simulink model "uz_mpc_6ph"  (R2021a)
settings: Solver=FixedStepDiscrete  StartTime=0.0  StopTime=3*1/f  RelTol=1e-3
values from neighbouring files (symbols this model uses):
  A = 1.0    (= 1)    [uz_6ph_pu_vsd_voltages_init.m]    (also in uz_mpc_6ph_init.m; uz_mpc_6ph_state_machine_init.m = 0.1)
  f = n_rpm/60.0*p    (= 250)    [uz_6ph_pu_vsd_voltages_init.m]    (also in uz_mpc_6ph_init.m; uz_mpc_6ph_state_machine_init.m = 83.3333333333)
  IB = sqrt(2)*IR    [uz_6ph_pu_vsd_voltages_init.m]    (also in uz_mpc_6ph_init.m; uz_mpc_6ph_state_machine_init.m)
  id_ref = 0.0    (= 0)    [uz_6ph_pu_vsd_voltages_init.m]    (also in uz_mpc_6ph_init.m; uz_mpc_6ph_state_machine_init.m)
  iq_ref = -10.0    (= -10)    [uz_6ph_pu_vsd_voltages_init.m]    (also in uz_mpc_6ph_init.m; uz_mpc_6ph_state_machine_init.m = 5)
  ix_ref = 0.0    (= 0)    [uz_6ph_pu_vsd_voltages_init.m]    (also in uz_mpc_6ph_init.m; uz_mpc_6ph_state_machine_init.m)
  iy_ref = 0.0    (= 0)    [uz_6ph_pu_vsd_voltages_init.m]    (also in uz_mpc_6ph_init.m; uz_mpc_6ph_state_machine_init.m)
  Ld_minus_Lq_over_LB = (Ld-Lq)/LB    [uz_6ph_pu_vsd_voltages_init.m]    (also in uz_mpc_6ph_init.m; uz_mpc_6ph_state_machine_init.m)
  Ld_over_LB = Ld/LB    [uz_6ph_pu_vsd_voltages_init.m]    (also in uz_mpc_6ph_init.m; uz_mpc_6ph_state_machine_init.m)
  Lq_over_LB = Lq/LB    [uz_6ph_pu_vsd_voltages_init.m]    (also in uz_mpc_6ph_init.m; uz_mpc_6ph_state_machine_init.m)
  omega_m = n_rpm*pi/30    (= 314.159265359)    [uz_6ph_pu_vsd_voltages_init.m]    (also in uz_mpc_6ph_init.m; uz_mpc_6ph_state_machine_init.m = 104.71975512)
  omegaB = nR*2*pi()/60*p    [uz_6ph_pu_vsd_voltages_init.m]    (also in uz_mpc_6ph_init.m; uz_mpc_6ph_state_machine_init.m)
  psi_pm_over_psiB = psi_pm/psiB    [uz_6ph_pu_vsd_voltages_init.m]    (also in uz_mpc_6ph_init.m; uz_mpc_6ph_state_machine_init.m)
  Rs_over_ZB = Rs/ZB    [uz_6ph_pu_vsd_voltages_init.m]    (also in uz_mpc_6ph_init.m; uz_mpc_6ph_state_machine_init.m)
  t_ADC = 1/f_ADC    (= 1e-05)    [uz_6ph_pu_vsd_voltages_init.m]    (also in uz_mpc_6ph_init.m; uz_mpc_6ph_state_machine_init.m; uz_typeconv_init.m)
  Ts_times_ZB_over_Ld = Ts*ZB/Ld    [uz_6ph_pu_vsd_voltages_init.m]    (also in uz_mpc_6ph_init.m; uz_mpc_6ph_state_machine_init.m)
  Ts_times_ZB_over_Lq = Ts*ZB/Lq    [uz_6ph_pu_vsd_voltages_init.m]    (also in uz_mpc_6ph_init.m; uz_mpc_6ph_state_machine_init.m)
  Ts_times_ZB_over_Lx = Ts*ZB/Lx    [uz_6ph_pu_vsd_voltages_init.m]    (also in uz_mpc_6ph_init.m; uz_mpc_6ph_state_machine_init.m)
  Ts_times_ZB_over_Ly = Ts*ZB/Ly    [uz_6ph_pu_vsd_voltages_init.m]    (also in uz_mpc_6ph_init.m; uz_mpc_6ph_state_machine_init.m)
  v_dc = 565.0    (= 565)    [uz_6ph_pu_vsd_voltages_init.m]    (also in uz_mpc_6ph_init.m; uz_mpc_6ph_state_machine_init.m)
  VB = sqrt(2/3)*VR    [uz_6ph_pu_vsd_voltages_init.m]    (also in uz_mpc_6ph_init.m; uz_mpc_6ph_state_machine_init.m)
libraries: fl_lib x7, nesl_utility x7, simulink x4, ee_lib x2, hdlsllib x1
(part 1 of 2)
settings Model: DataTypeOverride=Off  Creator=micha  LastModifiedBy=micha
settings SolverCC: AlgebraicLoopSolver=TrustRegion
settings DataIOCC: LimitDataPoints=on  SaveOutput=off  SaveTime=off
settings OptimizationCC: BlockReduction=off  ConditionallyExecuteInputs=off  DefaultParameterBehavior=Inlined  LifeSpan=inf
settings DebuggingCC: SignalRangeChecking=warning  AlgebraicLoopMsg=error  SingleTaskRateTransMsg=error  AllowSymbolicDim=off  StrictBusMsg=ErrorOnBusTreatedAsVector  SFUnexpectedBacktrackingDiag=warning  SFNoUnconditionalDefaultTransitionDiag=warning  SFExecutionAtInitializationDiag=none  SFMachineParentedDataDiag=warning  ArithmeticOperatorsInVariantConditions=warning
settings HardwareCC: ProdBitPerPointer=32  ProdBitPerSizeT=32  ProdBitPerPtrDiffT=32  ProdLargestAtomicFloat=None  ProdIntDivRoundTo=Undefined  ProdEndianess=Unspecified  ProdWordSize=32  ProdHWDeviceType=ASIC/FPGA->ASIC/FPGA  ProdEqTarget=off
settings SFSimCC: SimUseLocalCustomCode=off  CustomCodeUndefinedFunction=UseInterfaceOnly
settings RTWCC: RTWUseLocalCustomCode=off
settings CodeAppCC: StateflowObjectComments=on
settings GRTTargetCC: TargetLangStandard=C89/C90 (ANSI)
settings ConfigComp: CovScope=ReferencedModels  CovMetricSettings=dw  CovSaveCumulativeToWorkspaceVar=on  CovSaveSingleToWorkspaceVar=on  CovExternalEMLEnable=off  CovSFcnEnable=off

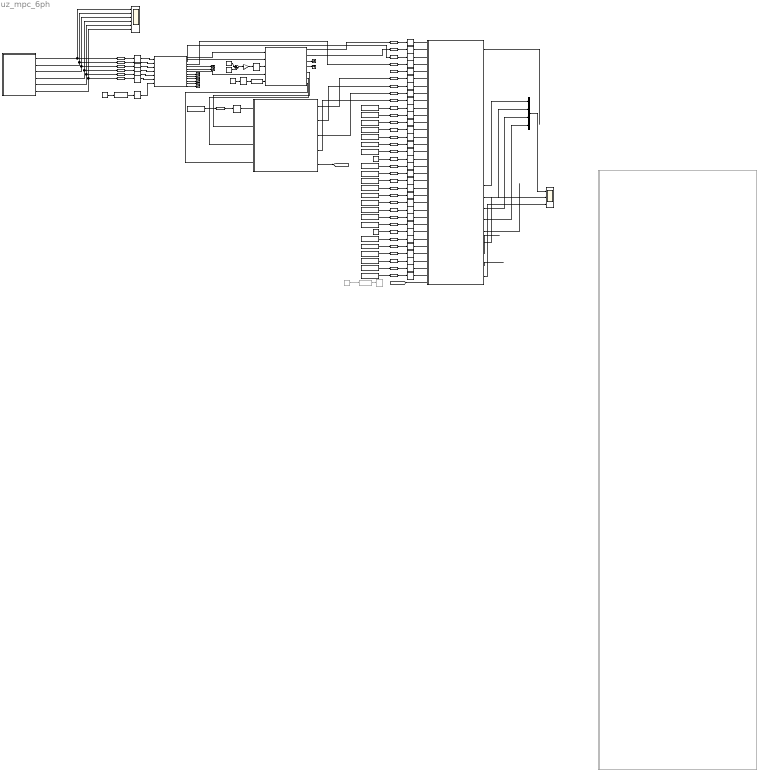
== system uz_mpc_6ph ==
  note: 0=AXI, 1=PL
  Constant : Constant  Value=5
  Constant1 : Constant  Value=0
  Constant10 : Constant  Value=psi_pm_over_psiB
  Constant11 : Constant  Value=2.5
  Constant12 : Constant  Value=0.0
  Constant{13..16} (4 alike) : Constant  Value=1.0
  Constant17 : Constant  Value=v_dc/VB
  Constant18 : Constant  Value=v_dc/VB
  Constant19 : Constant  Value=id_ref/IB
  Constant2 : Constant  Value=Rs_over_ZB
  Constant20 : Constant  Value=iq_ref/IB
  Constant21 : Constant  Value=ix_ref/IB
  Constant22 : Constant  Value=iy_ref/IB
  Constant23 : Constant  Value=omega_m/omegaB
  Constant24 : Constant  Value=2*pi
  Constant25 : Constant
  Constant26 : Constant  Value=v_dc/VB
  Constant3 : Constant  Value=Ts_times_ZB_over_Ld
  Constant4 : Constant  Value=Ts_times_ZB_over_Lq
  Constant5 : Constant  Value=Ts_times_ZB_over_Lx
  Constant6 : Constant  Value=Ts_times_ZB_over_Ly
  Constant7 : Constant  Value=Ld_over_LB
  Constant8 : Constant  Value=Lq_over_LB
  Constant9 : Constant  Value=Ld_minus_Lq_over_LB
  Data Type Conversion{,1,4,8..11} (7 alike) : DataTypeConversion  OutDataTypeStr=fixdt_type_xy_currents
  Data Type Conversion12 : DataTypeConversion  OutDataTypeStr=boolean
  Data Type Conversion13 : DataTypeConversion  OutDataTypeStr=fixdt_type_polepairs
  Data Type Conversion{14..18} (5 alike) : DataTypeConversion  OutDataTypeStr=fixdt_type_lambda
  Data Type Conversion19 : DataTypeConversion  OutDataTypeStr=fixdt_type_max_current
  Data Type Conversion2 : DataTypeConversion  OutDataTypeStr=fixdt_type_dq_currents
  Data Type Conversion{20..28} (9 alike) : DataTypeConversion  OutDataTypeStr=fixdt_type_constants
  Data Type Conversion29 : DataTypeConversion  OutDataTypeStr=fixdt_type_speed
  Data Type Conversion3 : DataTypeConversion  OutDataTypeStr=fixdt_type_dq_currents
  Data Type Conversion30 : DataTypeConversion  OutDataTypeStr=fixdt_type_voltage
  Data Type Conversion31 : DataTypeConversion  OutDataTypeStr=fixdt_type_voltage
  Data Type Conversion{32..36,38} (6 alike) : DataTypeConversion  OutDataTypeStr=fixdt_type_vsd
  Data Type Conversion37 : DataTypeConversion  OutDataTypeStr=boolean
  Data Type Conversion39 : DataTypeConversion  OutDataTypeStr=fixdt(1,18,14)
  Data Type Conversion40 : DataTypeConversion  OutDataTypeStr=fixdt_type_voltage
  Data Type Conversion{6..7,41..42} (4 alike) : DataTypeConversion  OutDataTypeStr=fixdt_type_dqxy_voltages
  Data Type Conversion5 : DataTypeConversion  Commented=on  OutDataTypeStr=boolean
  Gain : Gain  Gain=0.5
  Mux : Mux
  Pulse Generator : DiscretePulseGenerator  Commented=on  PulseType=Time based  Period=t_ADC  PulseWidth=5
  Pulse Generator1 : DiscretePulseGenerator  PulseType=Time based  Period=t_ADC  PulseWidth=5
  Rate Transition{1..2,4..43,58} (43 alike) : RateTransition  OutPortSampleTime=t_clock
  Rate Transition3 : RateTransition  Commented=on  OutPortSampleTime=t_clock
  Sawtooth Generator : SignalGenerator  WaveForm=sawtooth  Amplitude=2*pi  Frequency=2*pi*f  Units=rad/sec
  Scope : Scope  NumInputPorts=3
  Subsystem : Subsystem
  Sum : Sum  Inputs=|+-
  Terminator{,1..9} (10 alike) : Terminator
  natural values : Scope  NumInputPorts=6
  uz_6ph_pu_voltages_vsd : Subsystem
  uz_mpc_6ph : Subsystem  TreatAsAtomicUnit=on
  uz_mpc_current : MATLAB Function  Commented=on  TreatAsAtomicUnit=on  VariantControl=(default)
  uz_park_transformation : Subsystem  TreatAsAtomicUnit=on
  uz_vsd_6ph_30deg : Subsystem  TreatAsAtomicUnit=on
  wires:
  uz_mpc_6ph/1(G_T1) -> ?
  Pulse Generator/1 -> Data Type Conversion5/1
  Data Type Conversion5/1 -> Rate Transition3/1
  [calc_done] -> uz_mpc_6ph/34(trigger)  "trigger"
  Data Type Conversion/1 -> Rate Transition39/1
  Rate Transition39/1 -> uz_mpc_6ph/3(ix_pu)
  Data Type Conversion1/1 -> Rate Transition1/1
  Data Type Conversion2/1 -> Rate Transition2/1
  Data Type Conversion3/1 -> Rate Transition4/1
  Rate Transition1/1 -> uz_mpc_6ph/4(iy_pu)
  Rate Transition4/1 -> uz_mpc_6ph/2(iq_pu)
  Rate Transition2/1 -> uz_mpc_6ph/1(id_pu)
  Data Type Conversion4/1 -> Rate Transition5/1
  Rate Transition5/1 -> uz_mpc_6ph/5(angle_el)
  Data Type Conversion6/1 -> Rate Transition6/1
  Rate Transition6/1 -> uz_mpc_6ph/6(vd_pu)
  Data Type Conversion7/1 -> Rate Transition7/1
  Rate Transition7/1 -> uz_mpc_6ph/7(vq_pu)
  Rate Transition8/1 -> uz_mpc_6ph/11(id_ref_pu_AXI)
  Data Type Conversion8/1 -> Rate Transition8/1
  Rate Transition9/1 -> uz_mpc_6ph/12(iq_ref_pu_AXI)
  Data Type Conversion9/1 -> Rate Transition9/1
  Rate Transition10/1 -> uz_mpc_6ph/13(ix_ref_pu_AXI)
  Data Type Conversion10/1 -> Rate Transition10/1
  Rate Transition11/1 -> uz_mpc_6ph/14(iy_ref_pu_AXI)
  Data Type Conversion11/1 -> Rate Transition11/1
  Data Type Conversion12/1 -> Rate Transition12/1
  Rate Transition12/1 -> uz_mpc_6ph/17(v_dc_select_AXI)
  Data Type Conversion13/1 -> Rate Transition13/1
  Rate Transition13/1 -> uz_mpc_6ph/27(polepairs_AXI)
  Data Type Conversion14/1 -> Rate Transition14/1
  Rate Transition14/1 -> uz_mpc_6ph/29(lambda_u_AXI)
  Data Type Conversion15/1 -> Rate Transition15/1
  Rate Transition15/1 -> uz_mpc_6ph/30(lambda_d_AXI)
  Data Type Conversion16/1 -> Rate Transition16/1
  Rate Transition16/1 -> uz_mpc_6ph/31(lambda_q_AXI)
  Data Type Conversion17/1 -> Rate Transition17/1
  Rate Transition17/1 -> uz_mpc_6ph/32(lambda_x_AXI)
  Data Type Conversion18/1 -> Rate Transition18/1
  Rate Transition18/1 -> uz_mpc_6ph/33(lambda_y_AXI)
  Data Type Conversion19/1 -> Rate Transition19/1
  Rate Transition19/1 -> uz_mpc_6ph/28(max_current_pu_AXI)
  Rate Transition20/1 -> uz_mpc_6ph/15(v_dc_pu)
  Rate Transition21/1 -> uz_mpc_6ph/16(v_dc_pu_AXI)
  Rate Transition22/1 -> uz_mpc_6ph/18(Rs_over_ZB_AXI)
  Rate Transition28/1 -> uz_mpc_6ph/26(psi_pm_over_psiB_AXI)
  Rate Transition29/1 -> uz_mpc_6ph/19(Ts_times_ZB_over_Ld_AXI)
  Rate Transition25/1 -> uz_mpc_6ph/25(Ld_minus_Lq_over_LB_AXI)
  Rate Transition24/1 -> uz_mpc_6ph/22(Ts_times_ZB_over_Ly_AXI)
  Rate Transition26/1 -> uz_mpc_6ph/23(Ld_over_LB_AXI)
  Rate Transition30/1 -> uz_mpc_6ph/20(Ts_times_ZB_over_Lq_AXI)
  Rate Transition23/1 -> uz_mpc_6ph/21(Ts_times_ZB_over_Lx_AXI)
  Rate Transition27/1 -> uz_mpc_6ph/24(Lq_over_LB_AXI)
  Data Type Conversion20/1 -> Rate Transition22/1
  Data Type Conversion21/1 -> Rate Transition29/1
  Data Type Conversion22/1 -> Rate Transition30/1
  Data Type Conversion23/1 -> Rate Transition23/1
  Data Type Conversion24/1 -> Rate Transition24/1
  Data Type Conversion25/1 -> Rate Transition26/1
  Data Type Conversion26/1 -> Rate Transition27/1
  Data Type Conversion27/1 -> Rate Transition25/1
  Data Type Conversion28/1 -> Rate Transition28/1
  Data Type Conversion29/1 -> Rate Transition31/1
  Rate Transition31/1 -> uz_mpc_6ph/10(omega_m_pu)
  Data Type Conversion30/1 -> Rate Transition20/1
  Data Type Conversion31/1 -> Rate Transition21/1
  Constant/1 -> Data Type Conversion13/1
  Constant1/1 -> Data Type Conversion12/1
  Constant2/1 -> Data Type Conversion20/1
  Constant3/1 -> Data Type Conversion21/1
  Constant4/1 -> Data Type Conversion22/1
  Constant5/1 -> Data Type Conversion23/1
  Constant6/1 -> Data Type Conversion24/1
  Constant7/1 -> Data Type Conversion25/1
  Constant8/1 -> Data Type Conversion26/1
  Constant9/1 -> Data Type Conversion27/1
  Constant10/1 -> Data Type Conversion28/1
  Constant11/1 -> Data Type Conversion19/1
  Constant12/1 -> Data Type Conversion14/1
  Constant13/1 -> Data Type Conversion15/1
  Constant16/1 -> Data Type Conversion18/1
  Constant15/1 -> Data Type Conversion17/1
  Constant14/1 -> Data Type Conversion16/1
  Constant17/1 -> Data Type Conversion31/1
  Constant18/1 -> Data Type Conversion30/1
  Constant19/1 -> Data Type Conversion8/1
  Constant20/1 -> Data Type Conversion9/1
  Constant22/1 -> Data Type Conversion11/1
  Constant21/1 -> Data Type Conversion10/1
  Constant23/1 -> Data Type Conversion29/1
  Subsystem/1(output) -> natural values/1, Data Type Conversion32/1
  Rate Transition34/1 -> uz_vsd_6ph_30deg/4(a2)
  Subsystem/4(output3) -> Data Type Conversion35/1, natural values/4
  uz_vsd_6ph_30deg/3(x1) -> Data Type Conversion/1
  Data Type Conversion36/1 -> Rate Transition36/1
  Subsystem/2(output1) -> natural values/2, Data Type Conversion33/1
  Subsystem/5(output4) -> Data Type Conversion36/1, natural values/5
  Data Type Conversion37/1 -> Rate Transition58/1
  Data Type Conversion38/1 -> Rate Transition37/1
  Subsystem/6(output5) -> natural values/6, Data Type Conversion38/1
  Data Type Conversion34/1 -> Rate Transition33/1
  Data Type Conversion32/1 -> Rate Transition35/1
  Subsystem/3(output2) -> Data Type Conversion34/1, natural values/3
  Rate Transition32/1 -> uz_vsd_6ph_30deg/2(b1)
  Data Type Conversion35/1 -> Rate Transition34/1
  uz_vsd_6ph_30deg/5(z1) -> Terminator/1
  uz_vsd_6ph_30deg/1(alpha) -> uz_park_transformation/1(u1)
  Data Type Conversion33/1 -> Rate Transition32/1
  uz_vsd_6ph_30deg/6(z2) -> Terminator1/1
  uz_vsd_6ph_30deg/7(vsd_done) -> uz_park_transformation/4(trigger)
  uz_vsd_6ph_30deg/4(y1) -> Data Type Conversion1/1
  uz_vsd_6ph_30deg/2(beta) -> uz_park_transformation/2(u2)
  Rate Transition37/1 -> uz_vsd_6ph_30deg/6(c2)
  Pulse Generator1/1 -> Data Type Conversion37/1
  Rate Transition58/1 -> uz_vsd_6ph_30deg/7(pu_conv_valid)
  Rate Transition35/1 -> uz_vsd_6ph_30deg/1(a1)
  Rate Transition36/1 -> uz_vsd_6ph_30deg/5(b2)
  Rate Transition33/1 -> uz_vsd_6ph_30deg/3(c1)
  uz_6ph_pu_voltages_vsd/5(calc_done) -> [calc_done]  "calc_done"
  uz_park_transformation/1(y1) -> Data Type Conversion2/1
  uz_park_transformation/2(y2) -> Data Type Conversion3/1
  Sawtooth Generator/1 -> Sum/2
  Sum/1 -> Gain/1
  Constant24/1 -> Sum/1
  Gain/1 -> Rate Transition38/1
  Rate Transition38/1 -> uz_park_transformation/3(angle_el)
  Constant25/1 -> Rate Transition40/1
  Rate Transition40/1 -> Data Type Conversion39/1
  Data Type Conversion39/1 -> uz_park_transformation/5(factor_angle_el_AXI)
  Rate Transition41/1 -> uz_6ph_pu_voltages_vsd/1(v_DC_pu)
  Constant26/1 -> Data Type Conversion40/1
  Data Type Conversion40/1 -> Rate Transition41/1
  uz_park_transformation/5(sin) -> uz_6ph_pu_voltages_vsd/2(sin_angle)
  uz_park_transformation/6(cos) -> uz_6ph_pu_voltages_vsd/3(cos_angle)
  uz_park_transformation/7(calc_done) -> uz_6ph_pu_voltages_vsd/4(trigger)  "calc_done"
  Data Type Conversion41/1 -> Rate Transition42/1
  Data Type Conversion42/1 -> Rate Transition43/1
  Rate Transition42/1 -> uz_mpc_6ph/8(vx_pu)
  Rate Transition43/1 -> uz_mpc_6ph/9(vy_pu)
  uz_6ph_pu_voltages_vsd/1(pu_ud) -> Data Type Conversion6/1
  uz_6ph_pu_voltages_vsd/2(pu_uq) -> Data Type Conversion7/1
  uz_6ph_pu_voltages_vsd/3(pu_ux) -> Data Type Conversion41/1
  uz_6ph_pu_voltages_vsd/4(pu_uy) -> Data Type Conversion42/1
  uz_mpc_6ph/13(id_pred_pu_AXI) -> Mux/1
  uz_mpc_6ph/14(iq_pred_pu_AXI) -> Mux/2
  uz_mpc_6ph/15(ix_pred_pu_AXI) -> Mux/3
  uz_mpc_6ph/16(iy_pred_pu_AXI) -> Mux/4
  uz_mpc_6ph/17(T_el_pred_pu_AXI) -> ?
  uz_mpc_6ph/18(index_AXI) -> Scope/2
  uz_mpc_6ph/19(id_delay_pu_AXI) -> ?
  uz_mpc_6ph/20(iq_delay_pu_AXI) -> ?
  Mux/1 -> Scope/1
  uz_mpc_6ph/21(calc_done) -> Scope/3
  uz_vsd_6ph_30deg/8(alpha_AXI) -> Terminator2/1
  uz_vsd_6ph_30deg/9(beta_AXI) -> Terminator3/1
  uz_vsd_6ph_30deg/10(x_AXI) -> Terminator4/1
  uz_vsd_6ph_30deg/11(y_AXI) -> Terminator5/1
  uz_vsd_6ph_30deg/12(z1_AXI) -> Terminator6/1
  uz_vsd_6ph_30deg/13(z2_AXI) -> Terminator7/1
  uz_park_transformation/3(y1_AXI) -> Terminator8/1
  uz_park_transformation/4(y2_AXI) -> Terminator9/1

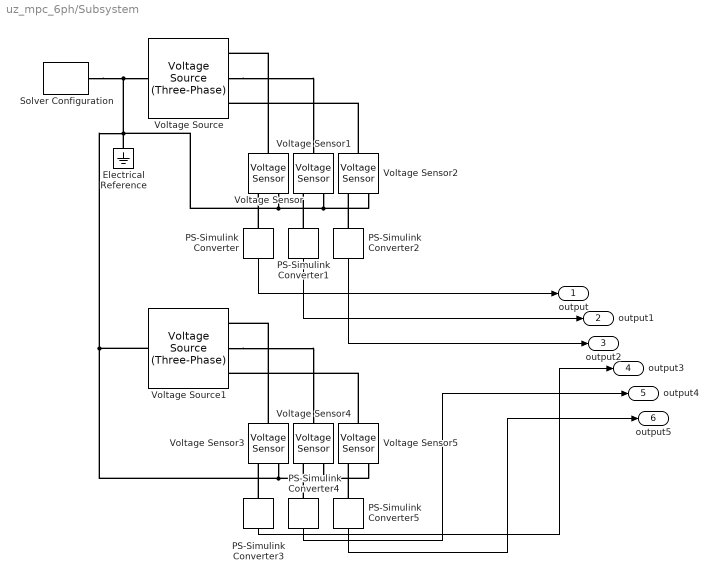
== system uz_mpc_6ph/Subsystem ==
  Electrical Reference : fl_lib/Electrical/Electrical Elements/Electrical Reference
  PS-Simulink Converter{,1..5} (6 alike) : nesl_utility/PS-Simulink Converter  PhysicalDomain=network_engine_domain  SubClassName=ps_output  LeftPortType=input  RightPortType=output  PseudoPeriodic=off  Frequencies=[]  Unit=1  AffineConversion=off
  Solver Configuration : nesl_utility/Solver Configuration  PhysicalDomain=network_engine_domain  SubClassName=solver  LeftPortType=input  RightPortType=generic  Tones=[]  Harmonics=[]  SimulateNoise=off  Profile=off  UseLocalSampling=off  EnableSwitchedLinearOptims=on  FrequencyDomain=off  UseCCode=off  RelTol=0.001  AbsTol=1e-06  MinStep=1e-09  ToWorkspace=off  RevertToSquareIcSolve=off  NumHomotopyIterations=100  PhasorMode=off  PhasorModeNumHarmonics=1  DoDC=off  ResidualTolerance=1e-09  UseLocalSolver=on  LocalSolverChoice=NE_BACKWARD_EULER_ADVANCER  LocalSolverSampleTime=1e-6  DoFixedCost=on  MaxNonlinIter=3  MaxModeIter=2  ComputeImpulses=off  ImpulseIterations=2  LinearAlgebra=Sparse  EquationFormulation=NE_TIME_EF  DelaysMemoryBudget=1024  AutomaticFiltering=on  FilteringTimeConstant=0.001  PartitionStorageMethod=AS_NEEDED  PartitionMemoryBudget=1024  PartitionMethod=FAST
  Voltage Sensor{,1..5} (6 alike) : fl_lib/Electrical/Electrical Sensors/Voltage Sensor
  Voltage Source : ee_lib/Sources/Voltage Source (Three-Phase)  vline_rms=A*sqrt(3)/sqrt(2) V  shift=0 deg  freq=f Hz  impedance_option=1  SShortCircuit=1e6 V*A  XR=15  R=0.01 Ohm  L=3.97e-4 H  G_parasitic=0 1/Ohm  harmonic_option=1  harmonic_orders=Harmonic_Orders  harmonic_ratios=Harmonic_Amplitudes  I_specify=off  I_priority=None  I=[ 0 0 0 ] A  I_nominal_specify=off  I_nominal_unit=A  I_nominal_value=1
      settings: SourceProductBaseCode=PS  InternalSimscapePortConfiguration="{\"Bottom\":[],\"Left\":[{\"id\":\"n\",\"label\":\"n\",\"type\":\"foundation.electrical.electrical\"}],\"Right\":[{\"id\":\"a\",\"label\":\"a\",\"type\":\"foundation.electrical.electrical\"},{\"id\":\"b\",\"label\":\"b\",\"type\":\"foundation.electrical.electrical\"},{\"id\":\"c\",\"label\":\"c\",\"type\":\"foundation.electrical.electrical\"}],\"Top\":[]}"
  Voltage Source1 : ee_lib/Sources/Voltage Source (Three-Phase)  vline_rms=A*sqrt(3)/sqrt(2) V  shift=-30 deg  freq=f Hz  impedance_option=1  SShortCircuit=1e6 V*A  XR=15  R=0.01 Ohm  L=3.97e-4 H  G_parasitic=0 1/Ohm  harmonic_option=1  harmonic_orders=Harmonic_Orders  harmonic_ratios=Harmonic_Amplitudes  I_specify=off  I_priority=None  I=[ 0 0 0 ] A  I_nominal_specify=off  I_nominal_unit=A  I_nominal_value=1
      settings: SourceProductBaseCode=PS  InternalSimscapePortConfiguration="{\"Bottom\":[],\"Left\":[{\"id\":\"n\",\"label\":\"n\",\"type\":\"foundation.electrical.electrical\"}],\"Right\":[{\"id\":\"a\",\"label\":\"a\",\"type\":\"foundation.electrical.electrical\"},{\"id\":\"b\",\"label\":\"b\",\"type\":\"foundation.electrical.electrical\"},{\"id\":\"c\",\"label\":\"c\",\"type\":\"foundation.electrical.electrical\"}],\"Top\":[]}"
  output : Outport
  output1 : Outport  Port=2
  output2 : Outport  Port=3
  output3 : Outport  Port=4
  output4 : Outport  Port=5
  output5 : Outport  Port=6
  wires:
  PS-Simulink Converter/1 -> output/1
  PS-Simulink Converter3/1 -> output3/1
  PS-Simulink Converter4/1 -> output4/1
  PS-Simulink Converter1/1 -> output1/1
  PS-Simulink Converter5/1 -> output5/1
  PS-Simulink Converter2/1 -> output2/1
  connections:
  Voltage Sensor5/RConn2 -- Solver Configuration/RConn1 -- Voltage Source/LConn1 -- Voltage Sensor2/RConn2 -- Voltage Sensor1/RConn2 -- Voltage Sensor/RConn2 -- Electrical Reference/LConn1 -- Voltage Source1/LConn1 -- Voltage Sensor3/RConn2 -- Voltage Sensor4/RConn2
  PS-Simulink Converter5/LConn1 -- Voltage Sensor5/RConn1
  PS-Simulink Converter1/LConn1 -- Voltage Sensor1/RConn1
  Voltage Sensor3/LConn1 -- Voltage Source1/RConn1
  PS-Simulink Converter/LConn1 -- Voltage Sensor/RConn1
  Voltage Source1/RConn2 -- Voltage Sensor4/LConn1
  Voltage Sensor5/LConn1 -- Voltage Source1/RConn3
  PS-Simulink Converter4/LConn1 -- Voltage Sensor4/RConn1
  Voltage Sensor2/LConn1 -- Voltage Source/RConn3
  PS-Simulink Converter2/LConn1 -- Voltage Sensor2/RConn1
  PS-Simulink Converter3/LConn1 -- Voltage Sensor3/RConn1
  Voltage Sensor/LConn1 -- Voltage Source/RConn1
  Voltage Source/RConn2 -- Voltage Sensor1/LConn1

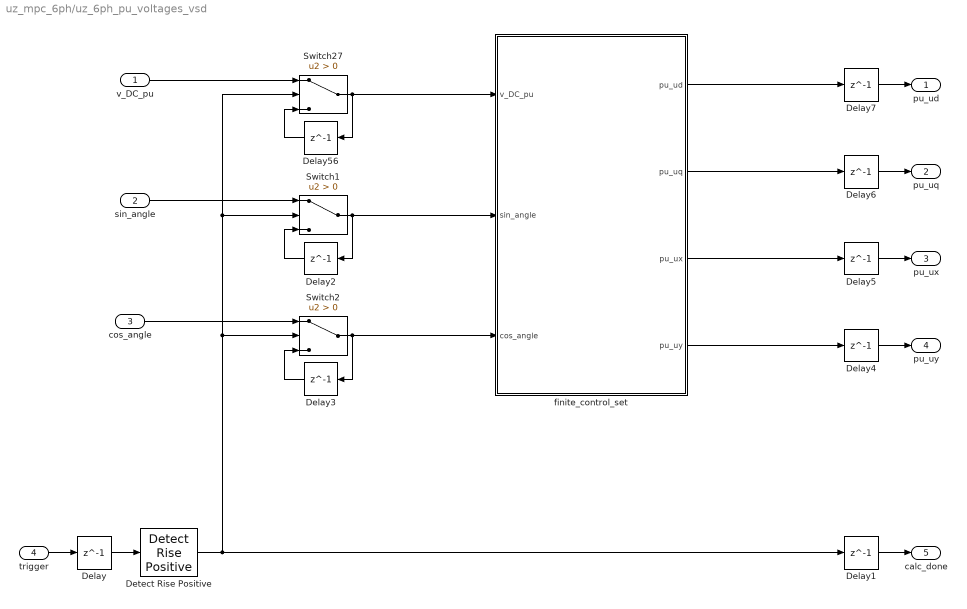
== system uz_mpc_6ph/uz_6ph_pu_voltages_vsd ==
  v_DC_pu : Inport
  sin_angle : Inport  Port=2
  cos_angle : Inport  Port=3
  trigger : Inport  Port=4
  Delay{,1..7,56} (9 alike) : Delay  DelayLength=1
  Detect Rise Positive : simulink/Logic and Bit Operations/Detect Rise Positive  vinit=0  OutDataTypeStr=boolean
  Switch1 : Switch  Criteria=u2 > Threshold
  Switch2 : Switch  Criteria=u2 > Threshold
  Switch27 : Switch  Criteria=u2 > Threshold
  finite_control_set : MATLAB Function  TreatAsAtomicUnit=on
  pu_ud : Outport
  pu_uq : Outport  Port=2
  pu_ux : Outport  Port=3
  pu_uy : Outport  Port=4
  calc_done : Outport  Port=5
  wires:
  finite_control_set/1(pu_ud) -> Delay7/1
  finite_control_set/2(pu_uq) -> Delay6/1
  finite_control_set/3(pu_ux) -> Delay5/1
  finite_control_set/4(pu_uy) -> Delay4/1
  trigger/1 -> Delay/1
  Delay/1 -> Detect Rise Positive/1
  Delay1/1 -> calc_done/1
  Delay56/1 -> Switch27/3
  v_DC_pu/1 -> Switch27/1
  Switch27/1 -> Delay56/1, finite_control_set/1(v_DC_pu)
  sin_angle/1 -> Switch1/1
  Delay2/1 -> Switch1/3
  Switch1/1 -> finite_control_set/2(sin_angle), Delay2/1
  cos_angle/1 -> Switch2/1
  Delay3/1 -> Switch2/3
  Switch2/1 -> finite_control_set/3(cos_angle), Delay3/1
  Detect Rise Positive/1 -> Switch2/2, Switch1/2, Switch27/2, Delay1/1
  Delay4/1 -> pu_uy/1
  Delay5/1 -> pu_ux/1
  Delay6/1 -> pu_uq/1
  Delay7/1 -> pu_ud/1

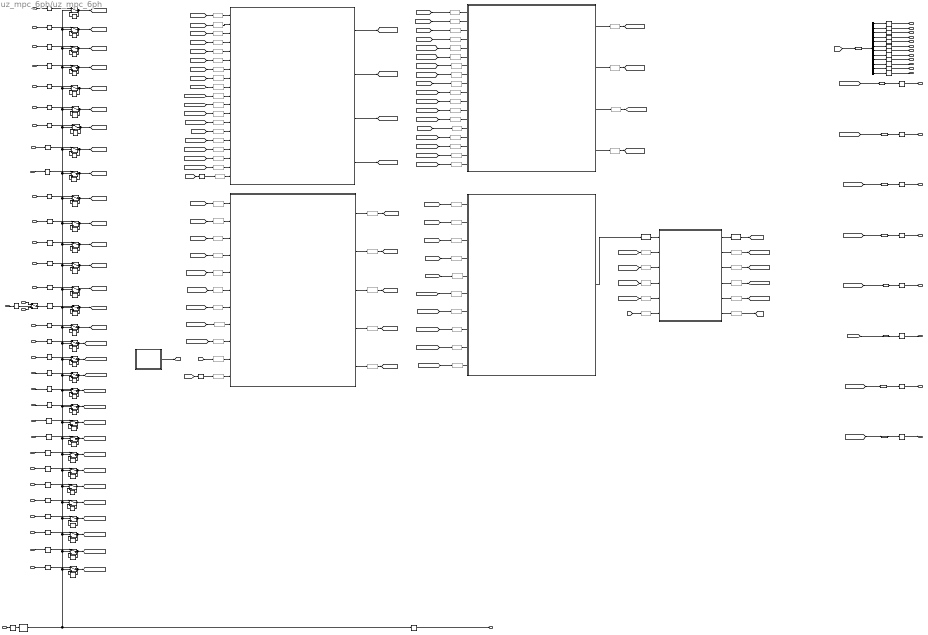
== system uz_mpc_6ph/uz_mpc_6ph ==
  note: 0=AXI, 1=PL
  id_pu : Inport
  iq_pu : Inport  Port=2
  ix_pu : Inport  Port=3
  iy_pu : Inport  Port=4
  angle_el : Inport  Port=5
  vd_pu : Inport  Port=6
  vq_pu : Inport  Port=7
  vx_pu : Inport  Port=8
  vy_pu : Inport  Port=9
  omega_m_pu : Inport  Port=10
  id_ref_pu_AXI : Inport  Port=11
  iq_ref_pu_AXI : Inport  Port=12
  ix_ref_pu_AXI : Inport  Port=13
  iy_ref_pu_AXI : Inport  Port=14
  v_dc_pu : Inport  Port=15
  v_dc_pu_AXI : Inport  Port=16
  v_dc_select_AXI : Inport  Port=17
  Rs_over_ZB_AXI : Inport  Port=18
  Ts_times_ZB_over_Ld_AXI : Inport  Port=19
  Ts_times_ZB_over_Lq_AXI : Inport  Port=20
  Ts_times_ZB_over_Lx_AXI : Inport  Port=21
  Ts_times_ZB_over_Ly_AXI : Inport  Port=22
  Ld_over_LB_AXI : Inport  Port=23
  Lq_over_LB_AXI : Inport  Port=24
  Ld_minus_Lq_over_LB_AXI : Inport  Port=25
  psi_pm_over_psiB_AXI : Inport  Port=26
  polepairs_AXI : Inport  Port=27
  max_current_pu_AXI : Inport  Port=28
  lambda_u_AXI : Inport  Port=29
  lambda_d_AXI : Inport  Port=30
  lambda_q_AXI : Inport  Port=31
  lambda_x_AXI : Inport  Port=32
  lambda_y_AXI : Inport  Port=33
  trigger : Inport  Port=34
  Data Type Conversion{,1..57,60..69,79..87} (77 alike) : DataTypeConversion  Commented=through  OutDataTypeStr=single
  Data Type Conversion58 : DataTypeConversion  OutDataTypeStr=fixdt(1,27,18)
  Data Type Conversion59 : DataTypeConversion  OutDataTypeStr=fixdt(0,18,0)
  Data Type Conversion{70..74,77..78} (7 alike) : DataTypeConversion  OutDataTypeStr=fixdt_type_dq_currents
  Data Type Conversion75 : DataTypeConversion  OutDataTypeStr=fixdt_type_polepairs
  Data Type Conversion76 : DataTypeConversion  OutDataTypeStr=boolean
  Delay{,1..73,76..86} (85 alike) : Delay  DelayLength=1
  Delay74 : Delay  DelayLength=1  InitialCondition=1
  Delay75 : Delay  DelayLength=1  InitialCondition=1
  Demux : Demux  Outputs=12
  Detect Rise Positive : simulink/Logic and Bit Operations/Detect Rise Positive  vinit=0  OutDataTypeStr=boolean
  FiniteControlSetSwitchingTable : MATLAB Function  TreatAsAtomicUnit=on
  MATLAB Function : MATLAB Function  TreatAsAtomicUnit=on
  Switch{,1..31} (32 alike) : Switch  Criteria=u2 > Threshold
  cost_function : MATLAB Function  TreatAsAtomicUnit=on
  delay_compensation : MATLAB Function  TreatAsAtomicUnit=on
  error_calculation : MATLAB Function  TreatAsAtomicUnit=on
  prediciton : MATLAB Function  TreatAsAtomicUnit=on
  G_T1 : Outport  VectorParamsAs1DForOutWhenUnconnected=off
  G_B1 : Outport  Port=2  VectorParamsAs1DForOutWhenUnconnected=off
  G_T2 : Outport  Port=3  VectorParamsAs1DForOutWhenUnconnected=off
  G_B2 : Outport  Port=4  VectorParamsAs1DForOutWhenUnconnected=off
  G_T3 : Outport  Port=5  VectorParamsAs1DForOutWhenUnconnected=off
  G_B3 : Outport  Port=6  VectorParamsAs1DForOutWhenUnconnected=off
  G_T4 : Outport  Port=7  VectorParamsAs1DForOutWhenUnconnected=off
  G_B4 : Outport  Port=8  VectorParamsAs1DForOutWhenUnconnected=off
  G_T5 : Outport  Port=9  VectorParamsAs1DForOutWhenUnconnected=off
  G_B5 : Outport  Port=10  VectorParamsAs1DForOutWhenUnconnected=off
  G_T6 : Outport  Port=11  VectorParamsAs1DForOutWhenUnconnected=off
  G_B6 : Outport  Port=12  VectorParamsAs1DForOutWhenUnconnected=off
  id_pred_pu_AXI : Outport  Port=13
  iq_pred_pu_AXI : Outport  Port=14
  ix_pred_pu_AXI : Outport  Port=15
  iy_pred_pu_AXI : Outport  Port=16
  T_el_pred_pu_AXI : Outport  Port=17
  index_AXI : Outport  Port=18
  id_delay_pu_AXI : Outport  Port=19
  iq_delay_pu_AXI : Outport  Port=20
  calc_done : Outport  Port=21
  wires:
  Delay/1 -> Detect Rise Positive/1
  trigger/1 -> Delay/1
  [Gates] -> Data Type Conversion76/1
  Delay61/1 -> G_T1/1
  Delay62/1 -> id_pred_pu_AXI/1
  [id_pred_idx_pu] -> Data Type Conversion70/1
  [iq_pred_idx_pu] -> Data Type Conversion71/1
  Delay63/1 -> iq_pred_pu_AXI/1
  [ix_pred_idx_pu] -> Data Type Conversion72/1
  Delay64/1 -> ix_pred_pu_AXI/1
  [iy_pred_idx_pu] -> Data Type Conversion73/1
  Delay65/1 -> iy_pred_pu_AXI/1
  [T_el_pred_pu] -> Data Type Conversion74/1
  Delay66/1 -> T_el_pred_pu_AXI/1
  [index] -> Data Type Conversion75/1
  Delay67/1 -> index_AXI/1
  [id_delay_pu] -> Data Type Conversion77/1
  Delay68/1 -> id_delay_pu_AXI/1
  [iq_delay_pu] -> Data Type Conversion78/1
  Delay69/1 -> iq_delay_pu_AXI/1
  Switch30/1 -> Delay70/1, [vx_pu]
  Delay70/1 -> Switch30/3
  Delay72/1 -> Switch31/3
  vy_pu/1 -> Delay73/1
  Delay41/1 -> Switch20/1
  Switch18/1 -> Delay38/1, [Lq_over_LB_AXI]
  Delay10/1 -> Switch4/1
  Switch19/1 -> [psi_pm_over_psiB_AXI], Delay40/1
  psi_pm_over_psiB_AXI/1 -> Delay39/1
  Delay13/1 -> Switch5/3
  v_dc_pu/1 -> Switch11/1
  Delay40/1 -> Switch19/3
  Delay39/1 -> Switch19/1
  Delay38/1 -> Switch18/3
  Delay30/1 -> Switch14/3
  Delay35/1 -> Switch17/1
  Delay36/1 -> Switch17/3
  Delay32/1 -> Switch15/3
  Ts_times_ZB_over_Ld_AXI/1 -> Delay27/1
  Ts_times_ZB_over_Lq_AXI/1 -> Delay29/1
  Rs_over_ZB_AXI/1 -> Delay25/1
  Switch7/1 -> [iq_ref_pu_AXI], Delay17/1
  Ld_over_LB_AXI/1 -> Delay35/1
  Switch16/1 -> Delay34/1, [Ts_times_ZB_over_Ly_AXI]
  Switch15/1 -> [Ts_times_ZB_over_Lx_AXI], Delay32/1
  Delay34/1 -> Switch16/3
  Lq_over_LB_AXI/1 -> Delay37/1
  Switch4/1 -> [angle_el], Delay11/1
  ix_ref_pu_AXI/1 -> Delay18/1
  Delay28/1 -> Switch13/3
  omega_m_pu/1 -> Delay12/1
  Delay27/1 -> Switch13/1
  Delay6/1 -> Switch2/1
  Switch9/1 -> [iy_ref_pu_AXI], Delay21/1
  Switch11/1 -> Delay22/1
  Delay17/1 -> Switch7/3
  Switch5/1 -> [omega_m_pu], Delay13/1
  Switch8/1 -> [ix_ref_pu_AXI], Delay19/1
  iy_pu/1 -> Delay8/1
  iq_pu/1 -> Delay4/1
  v_dc_select_AXI/1 -> Delay24/1
  Switch3/1 -> [iy_pu], Delay9/1
  Switch2/1 -> [ix_pu], Delay7/1
  Delay5/1 -> Switch1/3
  Delay4/1 -> Switch1/1
  Switch13/1 -> [Ts_times_ZB_over_Ld_AXI], Delay28/1
  Switch1/1 -> [iq_pu], Delay5/1
  Delay3/1 -> Switch/3
  Delay11/1 -> Switch4/3
  Delay52/1 -> Switch27/1
  Delay19/1 -> Switch8/3
  Delay12/1 -> Switch5/1
  v_dc_pu_AXI/1 -> Switch11/3
  Delay60/1 -> Switch29/1
  lambda_u_AXI/1 -> Delay47/1
  angle_el/1 -> Delay10/1
  Delay73/1 -> Switch31/1
  Delay57/1 -> Switch28/3
  Switch12/1 -> [Rs_over_ZB_AXI], Delay26/1
  Delay55/1 -> Switch26/3
  Switch24/1 -> [lambda_d_AXI], Delay53/1
  Delay9/1 -> Switch3/3
  Delay56/1 -> Switch27/3
  Delay53/1 -> Switch24/3
  Delay15/1 -> Switch6/3
  Delay54/1 -> Switch25/3
  Delay45/1 -> Switch22/1
  Delay51/1 -> Switch26/1
  Delay49/1 -> Switch24/1
  Switch10/1 -> [v_dc_pu], Delay23/1
  Switch21/1 -> [polepairs_AXI], Delay44/1
  Switch14/1 -> [Ts_times_ZB_over_Lq_AXI], Delay30/1
  Switch23/1 -> [lambda_u_AXI], Delay48/1
  Delay46/1 -> Switch22/3
  Ld_minus_Lq_over_LB_AXI/1 -> Delay41/1
  Ts_times_ZB_over_Ly_AXI/1 -> Delay33/1
  Switch22/1 -> [max_current_pu_AXI], Delay46/1
  Delay43/1 -> Switch21/1
  Delay47/1 -> Switch23/1
  Delay2/1 -> Switch/1
  Delay14/1 -> Switch6/1
  Delay48/1 -> Switch23/3
  Switch28/1 -> [vd_pu], Delay57/1
  Switch6/1 -> Delay15/1, [id_ref_pu_AXI]
  Delay7/1 -> Switch2/3
  Switch17/1 -> Delay36/1, [Ld_over_LB_AXI]
  Delay20/1 -> Switch9/1
  id_ref_pu_AXI/1 -> Delay14/1
  max_current_pu_AXI/1 -> Delay45/1
  Delay29/1 -> Switch14/1
  Delay59/1 -> Switch28/1
  Delay18/1 -> Switch8/1
  lambda_y_AXI/1 -> Delay52/1
  Delay25/1 -> Switch12/1
  Delay31/1 -> Switch15/1
  Detect Rise Positive/1 -> Switch27/2, Switch26/2, Switch25/2, Switch24/2, Switch23/2, Switch31/2, Switch30/2, Switch29/2, Switch28/2, Switch4/2, Switch3/2, Switch2/2, Switch1/2, Switch/2, Switch5/2, Switch6/2, Switch7/2, Switch8/2, Switch9/2, Switch10/2, Switch12/2, Switch13/2, Switch14/2, Switch15/2, Switch16/2, Switch17/2, Switch18/2, Switch20/2, Switch19/2, Switch21/2, Switch22/2, Delay1/1
  Delay16/1 -> Switch7/1
  Ts_times_ZB_over_Lx_AXI/1 -> Delay31/1
  Delay24/1 -> Switch11/2
  Delay22/1 -> Switch10/1
  Delay58/1 -> Switch29/3
  Delay33/1 -> Switch16/1
  Delay26/1 -> Switch12/3
  Delay37/1 -> Switch18/1
  Switch31/1 -> Delay72/1, [vy_pu]
  Switch20/1 -> [Ld_minus_Lq_over_LB_AXI], Delay42/1
  id_pu/1 -> Delay2/1
  iq_ref_pu_AXI/1 -> Delay16/1
  Switch/1 -> [id_pu], Delay3/1
  iy_ref_pu_AXI/1 -> Delay20/1
  Delay8/1 -> Switch3/1
  Delay50/1 -> Switch25/1
  ix_pu/1 -> Delay6/1
  Delay42/1 -> Switch20/3
  Switch29/1 -> [vq_pu], Delay58/1
  Delay71/1 -> Switch30/1
  lambda_d_AXI/1 -> Delay49/1
  vx_pu/1 -> Delay71/1
  Delay44/1 -> Switch21/3
  vq_pu/1 -> Delay60/1
  Delay21/1 -> Switch9/3
  Delay23/1 -> Switch10/3
  Switch25/1 -> [lambda_q_AXI], Delay54/1
  lambda_x_AXI/1 -> Delay51/1
  polepairs_AXI/1 -> Delay43/1
  Switch26/1 -> Delay55/1, [lambda_x_AXI]
  lambda_q_AXI/1 -> Delay50/1
  Switch27/1 -> Delay56/1, [lambda_y_AXI]
  vd_pu/1 -> Delay59/1
  prediciton/4(iy_pred_pu) -> Data Type Conversion87/1
  prediciton/2(iq_pred_pu) -> Data Type Conversion85/1
  prediciton/3(ix_pred_pu) -> Data Type Conversion86/1
  prediciton/1(id_pred_pu) -> Data Type Conversion84/1
  [vd_pu] -> Data Type Conversion/1
  Data Type Conversion/1 -> delay_compensation/1(vd_pu)
  [vq_pu] -> Data Type Conversion1/1
  Data Type Conversion1/1 -> delay_compensation/2(vq_pu)
  [vx_pu] -> Data Type Conversion2/1
  Data Type Conversion2/1 -> delay_compensation/3(vx_pu)
  [vy_pu] -> Data Type Conversion3/1
  Data Type Conversion4/1 -> delay_compensation/5(id_k_pu)
  [iq_pu] -> Data Type Conversion5/1
  Data Type Conversion5/1 -> delay_compensation/6(iq_k_pu)
  Data Type Conversion3/1 -> delay_compensation/4(vy_pu)
  [id_pu] -> Data Type Conversion4/1
  Data Type Conversion7/1 -> delay_compensation/8(iy_k_pu)
  [Ts_times_ZB_over_Ld_AXI] -> Data Type Conversion9/1
  [Ts_times_ZB_over_Lx_AXI] -> Data Type Conversion11/1
  Data Type Conversion11/1 -> delay_compensation/12(Ts_times_ZB_over_Lx)
  [Ts_times_ZB_over_Lq_AXI] -> Data Type Conversion10/1
  [ix_pu] -> Data Type Conversion6/1
  [omega_m_pu] -> Data Type Conversion8/1
  Data Type Conversion9/1 -> delay_compensation/10(Ts_times_ZB_over_Ld)
  Data Type Conversion10/1 -> delay_compensation/11(Ts_times_ZB_over_Lq)
  Data Type Conversion8/1 -> delay_compensation/9(omega_m_pu)
  Data Type Conversion6/1 -> delay_compensation/7(ix_k_pu)
  [iy_pu] -> Data Type Conversion7/1
  [psi_pm_over_psiB_AXI] -> Data Type Conversion12/1
  [Lq_over_LB_AXI] -> Data Type Conversion17/1
  Data Type Conversion15/1 -> delay_compensation/14(Rs_over_ZB)
  Data Type Conversion16/1 -> delay_compensation/15(Ld_over_LB)
  Data Type Conversion13/1 -> delay_compensation/18(polepairs)
  [Ld_over_LB_AXI] -> Data Type Conversion16/1
  [polepairs_AXI] -> Data Type Conversion13/1
  [Rs_over_ZB_AXI] -> Data Type Conversion15/1
  Data Type Conversion17/1 -> delay_compensation/16(Lq_over_LB)
  Data Type Conversion12/1 -> delay_compensation/17(psi_pm_over_psiB)
  Data Type Conversion14/1 -> delay_compensation/13(Ts_times_ZB_over_Ly)
  [Ts_times_ZB_over_Ly_AXI] -> Data Type Conversion14/1
  [Ts_times_ZB_over_Lq_AXI] -> Data Type Conversion20/1
  Data Type Conversion34/1 -> prediciton/9(omega_m_pu)
  [ix_delay_pu] -> Data Type Conversion32/1
  Data Type Conversion32/1 -> prediciton/7(ix_k_pu)
  Data Type Conversion20/1 -> prediciton/11(Ts_times_ZB_over_Lq)
  Data Type Conversion21/1 -> prediciton/12(Ts_times_ZB_over_Lx)
  [iy_delay_pu] -> Data Type Conversion33/1
  Data Type Conversion35/1 -> prediciton/10(Ts_times_ZB_over_Ld)
  [omega_m_pu] -> Data Type Conversion34/1
  [Ts_times_ZB_over_Lx_AXI] -> Data Type Conversion21/1
  [vy_pu] -> Data Type Conversion29/1
  [id_delay_pu] -> Data Type Conversion30/1
  Data Type Conversion33/1 -> prediciton/8(iy_k_pu)
  [vd_pu] -> Data Type Conversion18/1
  [Ld_over_LB_AXI] -> Data Type Conversion25/1
  Data Type Conversion29/1 -> prediciton/4(vy_pu)
  Data Type Conversion30/1 -> prediciton/5(id_k_pu)
  Data Type Conversion22/1 -> prediciton/17(psi_pm_over_psiB)
  Data Type Conversion26/1 -> prediciton/16(Lq_over_LB)
  Data Type Conversion23/1 -> prediciton/18(polepairs)
  Data Type Conversion18/1 -> prediciton/1(vd_pu)
  Data Type Conversion24/1 -> prediciton/13(Ts_times_ZB_over_Ly)
  Data Type Conversion25/1 -> prediciton/15(Ld_over_LB)
  [polepairs_AXI] -> Data Type Conversion23/1
  Data Type Conversion19/1 -> prediciton/2(vq_pu)
  [Ts_times_ZB_over_Ld_AXI] -> Data Type Conversion35/1
  [iq_delay_pu] -> Data Type Conversion31/1
  [Lq_over_LB_AXI] -> Data Type Conversion26/1
  [vx_pu] -> Data Type Conversion28/1
  Data Type Conversion28/1 -> prediciton/3(vx_pu)
  [Ts_times_ZB_over_Ly_AXI] -> Data Type Conversion24/1
  Data Type Conversion31/1 -> prediciton/6(iq_k_pu)
  [vq_pu] -> Data Type Conversion19/1
  [psi_pm_over_psiB_AXI] -> Data Type Conversion22/1
  [Rs_over_ZB_AXI] -> Data Type Conversion37/1
  Data Type Conversion37/1 -> prediciton/14(Rs_over_ZB)
  Data Type Conversion38/1 -> delay_compensation/19(index)
  delay_compensation/1(id_delay_pu) -> [id_delay_pu]
  delay_compensation/2(iq_delay_pu) -> [iq_delay_pu]
  delay_compensation/3(ix_delay_pu) -> [ix_delay_pu]
  delay_compensation/4(iy_delay_pu) -> [iy_delay_pu]
  Data Type Conversion49/1 -> error_calculation/9(max_current_pu)
  [ix_pred_pu] -> Data Type Conversion47/1
  Data Type Conversion47/1 -> error_calculation/7(ix_pred_pu)
  Data Type Conversion40/1 -> error_calculation/11(index_prev)
  [iy_pred_pu] -> Data Type Conversion48/1
  Data Type Conversion50/1 -> error_calculation/10(G)
  [max_current_pu_AXI] -> Data Type Conversion49/1
  Delay74/1 -> Data Type Conversion40/1
  Data Type Conversion36/1 -> error_calculation/2(iq_ref_pu)
  [G] -> Data Type Conversion50/1
  [iy_ref_pu_AXI] -> Data Type Conversion44/1
  [iq_pred_pu] -> Data Type Conversion46/1
  [id_pred_pu] -> Data Type Conversion45/1
  Data Type Conversion48/1 -> error_calculation/8(iy_pred_pu)
  [id_ref_pu_AXI] -> Data Type Conversion27/1
  [ix_ref_pu_AXI] -> Data Type Conversion43/1
  Data Type Conversion44/1 -> error_calculation/4(iy_ref_pu)
  Data Type Conversion45/1 -> error_calculation/5(id_pred_pu)
  Data Type Conversion43/1 -> error_calculation/3(ix_ref_pu)
  Data Type Conversion27/1 -> error_calculation/1(id_ref_pu)
  Data Type Conversion46/1 -> error_calculation/6(iq_pred_pu)
  [iq_ref_pu_AXI] -> Data Type Conversion36/1
  error_calculation/1(e_id_pu) -> Data Type Conversion79/1
  error_calculation/2(e_iq_pu) -> Data Type Conversion80/1
  error_calculation/3(e_ix_pu) -> Data Type Conversion81/1
  error_calculation/4(e_iy_pu) -> Data Type Conversion82/1
  error_calculation/5(delta_u) -> Data Type Conversion83/1
  [lambda_q_AXI] -> Data Type Conversion54/1
  Data Type Conversion54/1 -> cost_function/7(lambda_q)
  Data Type Conversion53/1 -> cost_function/6(lambda_d)
  [e_id_pu] -> Data Type Conversion55/1
  Data Type Conversion51/1 -> cost_function/9(lambda_y)
  [lambda_x_AXI] -> Data Type Conversion42/1
  Data Type Conversion56/1 -> cost_function/5(delta_u)
  Data Type Conversion41/1 -> cost_function/3(e_ix_pu)
  [e_iq_pu] -> Data Type Conversion39/1
  Data Type Conversion39/1 -> cost_function/2(e_iq_pu)
  Data Type Conversion55/1 -> cost_function/1(e_id_pu)
  [e_iy_pu] -> Data Type Conversion52/1
  Data Type Conversion52/1 -> cost_function/4(e_iy_pu)
  [e_ix_pu] -> Data Type Conversion41/1
  [delta_u] -> Data Type Conversion56/1
  [lambda_d_AXI] -> Data Type Conversion53/1
  [lambda_y_AXI] -> Data Type Conversion51/1
  Data Type Conversion42/1 -> cost_function/8(lambda_x)
  [lambda_u_AXI] -> Data Type Conversion57/1
  Data Type Conversion57/1 -> cost_function/10(lambda_u)
  cost_function/1(costs) -> Data Type Conversion58/1
  Data Type Conversion58/1 -> MATLAB Function/1(costs)
  MATLAB Function/1(index) -> Data Type Conversion59/1
  Data Type Conversion59/1 -> [index]
  Data Type Conversion60/1 -> MATLAB Function/6(G)
  [G] -> Data Type Conversion60/1
  FiniteControlSetSwitchingTable/1(G) -> [G]
  MATLAB Function/6(Gates) -> Data Type Conversion61/1
  Data Type Conversion61/1 -> [Gates]
  [index] -> Delay74/1
  Data Type Conversion62/1 -> MATLAB Function/2(id_pred_pu)
  Data Type Conversion64/1 -> MATLAB Function/4(ix_pred_pu)
  Data Type Conversion63/1 -> MATLAB Function/3(iq_pred_pu)
  Data Type Conversion65/1 -> MATLAB Function/5(iy_pred_pu)
  [iq_pred_pu] -> Data Type Conversion63/1
  [id_pred_pu] -> Data Type Conversion62/1
  [iy_pred_pu] -> Data Type Conversion65/1
  [ix_pred_pu] -> Data Type Conversion64/1
  Data Type Conversion66/1 -> [id_pred_idx_pu]
  MATLAB Function/2(id_pred_idx_pu) -> Data Type Conversion66/1
  Data Type Conversion68/1 -> [ix_pred_idx_pu]
  MATLAB Function/4(ix_pred_idx_pu) -> Data Type Conversion68/1
  Data Type Conversion67/1 -> [iq_pred_idx_pu]
  MATLAB Function/3(iq_pred_idx_pu) -> Data Type Conversion67/1
  MATLAB Function/5(iy_pred_idx_pu) -> Data Type Conversion69/1
  Data Type Conversion69/1 -> [iy_pred_idx_pu]
  Delay75/1 -> Data Type Conversion38/1
  [index] -> Delay75/1
  Delay1/1 -> calc_done/1
  Data Type Conversion70/1 -> Delay62/1
  Data Type Conversion71/1 -> Delay63/1
  Data Type Conversion72/1 -> Delay64/1
  Data Type Conversion73/1 -> Delay65/1
  Data Type Conversion74/1 -> Delay66/1
  Data Type Conversion75/1 -> Delay67/1
  Data Type Conversion76/1 -> Demux/1
  Data Type Conversion77/1 -> Delay68/1
  Data Type Conversion78/1 -> Delay69/1
  Data Type Conversion79/1 -> [e_id_pu]
  Data Type Conversion80/1 -> [e_iq_pu]
  Data Type Conversion81/1 -> [e_ix_pu]
  Data Type Conversion82/1 -> [e_iy_pu]
  Data Type Conversion83/1 -> [delta_u]
  Data Type Conversion84/1 -> [id_pred_pu]
  Data Type Conversion85/1 -> [iq_pred_pu]
  Data Type Conversion86/1 -> [ix_pred_pu]
  Data Type Conversion87/1 -> [iy_pred_pu]
  Delay76/1 -> G_B1/1
  Delay78/1 -> G_B2/1
  Delay77/1 -> G_T2/1
  Delay80/1 -> G_B3/1
  Delay79/1 -> G_T3/1
  Demux/1 -> Delay61/1
  Demux/2 -> Delay76/1
  Demux/3 -> Delay77/1
  Demux/4 -> Delay78/1
  Demux/5 -> Delay79/1
  Demux/6 -> Delay80/1
  Delay82/1 -> G_B4/1
  Delay83/1 -> G_T5/1
  Delay84/1 -> G_B5/1
  Delay86/1 -> G_B6/1
  Delay85/1 -> G_T6/1
  Delay81/1 -> G_T4/1
  Demux/7 -> Delay81/1
  Demux/8 -> Delay82/1
  Demux/9 -> Delay83/1
  Demux/10 -> Delay84/1
  Demux/11 -> Delay85/1
  Demux/12 -> Delay86/1

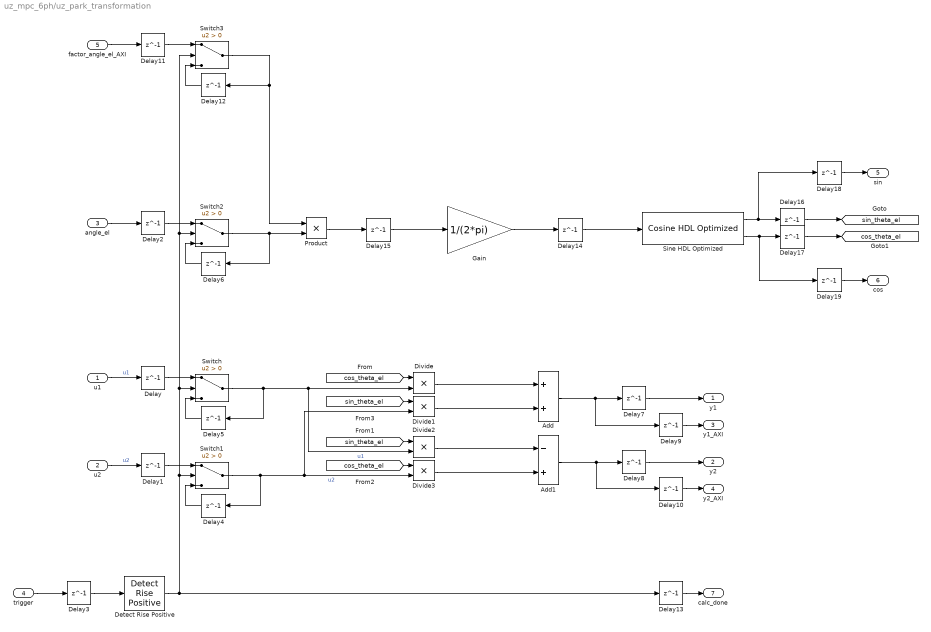
== system uz_mpc_6ph/uz_park_transformation ==
  u1 : Inport
  u2 : Inport  Port=2
  angle_el : Inport  Port=3
  trigger : Inport  Port=4
  factor_angle_el_AXI : Inport  Port=5
  Add : Sum  OutDataTypeStr=fixdt(1,27,16)
  Add1 : Sum  Inputs=-+  OutDataTypeStr=fixdt(1,27,16)
  Delay{,1..19} (20 alike) : Delay  DelayLength=1
  Detect Rise Positive : simulink/Logic and Bit Operations/Detect Rise Positive  vinit=0  OutDataTypeStr=boolean
  Divide{,1..3} (4 alike) : Product  Inputs=**  OutDataTypeStr=fixdt(1,27,16)
  Gain : Gain  Gain=1/(2*pi)  OutDataTypeStr=fixdt(1,18,16)
  Product : Product  OutDataTypeStr=fixdt(1,18,14)
  Sine HDL Optimized : hdlsllib/Lookup Tables/Cosine HDL Optimized  OutputFormula=sin(2*pi*u) and cos(2*pi*u)  NumDataPoints=256  TableDataTypeStr=fixdt(0,17,16)  SimulateLUTROMDelay=off
      settings: SourceProductBaseCode=SL
  Switch{,1..3} (4 alike) : Switch  Criteria=u2 > Threshold
  y1 : Outport  VectorParamsAs1DForOutWhenUnconnected=off
  y2 : Outport  Port=2  VectorParamsAs1DForOutWhenUnconnected=off
  y1_AXI : Outport  Port=3  VectorParamsAs1DForOutWhenUnconnected=off
  y2_AXI : Outport  Port=4  VectorParamsAs1DForOutWhenUnconnected=off
  sin : Outport  Port=5  VectorParamsAs1DForOutWhenUnconnected=off
  cos : Outport  Port=6  VectorParamsAs1DForOutWhenUnconnected=off
  calc_done : Outport  Port=7  VectorParamsAs1DForOutWhenUnconnected=off
  tag scope: cos_theta_el=global, sin_theta_el=global
  wires:
  Switch1/1 -> Delay4/1, Divide1/2, Divide3/2  "u2"
  Divide2/1 -> Add1/1
  Divide3/1 -> Add1/2
  [cos_theta_el] -> Divide3/1
  Switch/1 -> Divide2/2, Divide/2, Delay5/1  "u1"
  [sin_theta_el] -> Divide2/1
  Divide1/1 -> Add/2
  [cos_theta_el] -> Divide/1
  [sin_theta_el] -> Divide1/1
  Add/1 -> Delay9/1, Delay7/1
  Add1/1 -> Delay10/1, Delay8/1
  Divide/1 -> Add/1
  angle_el/1 -> Delay2/1
  Sine HDL Optimized/2 -> Delay19/1, Delay17/1
  Sine HDL Optimized/1 -> Delay18/1, Delay16/1
  Gain/1 -> Delay14/1
  u1/1 -> Delay/1  "u1"
  u2/1 -> Delay1/1  "u2"
  Delay/1 -> Switch/1
  Delay1/1 -> Switch1/1
  Delay2/1 -> Switch2/1
  trigger/1 -> Delay3/1
  Delay4/1 -> Switch1/3
  Delay5/1 -> Switch/3
  Delay6/1 -> Switch2/3
  Delay7/1 -> y1/1
  Delay8/1 -> y2/1
  Delay9/1 -> y1_AXI/1
  Delay10/1 -> y2_AXI/1
  Switch2/1 -> Product/2, Delay6/1
  Switch3/1 -> Product/1, Delay12/1
  factor_angle_el_AXI/1 -> Delay11/1
  Detect Rise Positive/1 -> Delay13/1, Switch1/2, Switch/2, Switch3/2, Switch2/2
  Delay12/1 -> Switch3/3
  Delay11/1 -> Switch3/1
  Product/1 -> Delay15/1
  Delay3/1 -> Detect Rise Positive/1
  Delay13/1 -> calc_done/1
  Delay15/1 -> Gain/1
  Delay14/1 -> Sine HDL Optimized/1
  Delay16/1 -> [sin_theta_el]
  Delay17/1 -> [cos_theta_el]
  Delay18/1 -> sin/1
  Delay19/1 -> cos/1

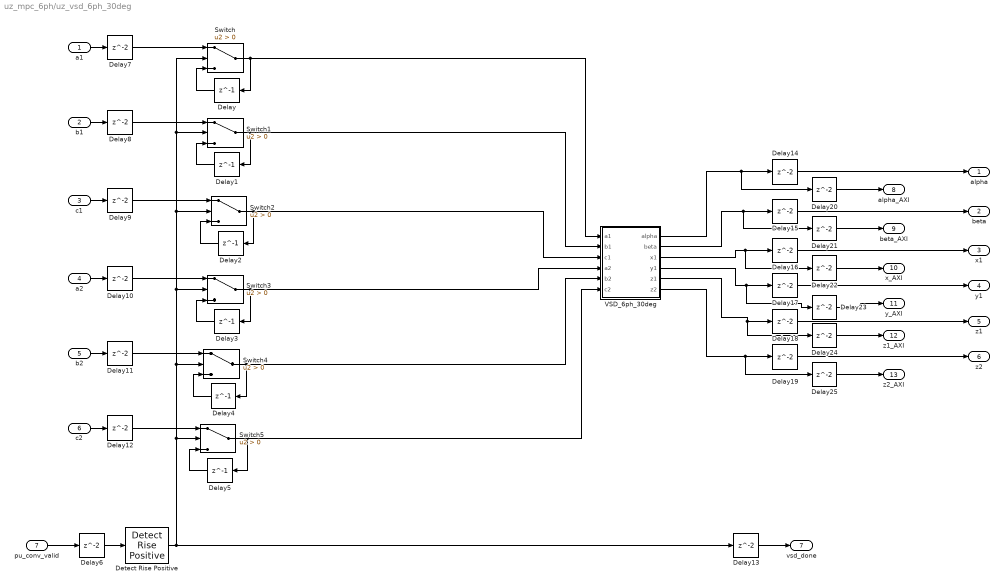
== system uz_mpc_6ph/uz_vsd_6ph_30deg ==
  a1 : Inport
  b1 : Inport  Port=2
  c1 : Inport  Port=3
  a2 : Inport  Port=4
  b2 : Inport  Port=5
  c2 : Inport  Port=6
  pu_conv_valid : Inport  Port=7
  Delay{,1..5} (6 alike) : Delay  DelayLength=1
  Delay{6..25} (20 alike) : Delay
  Detect Rise Positive : simulink/Logic and Bit Operations/Detect Rise Positive  vinit=0  OutDataTypeStr=boolean
  Switch{,1..5} (6 alike) : Switch  Criteria=u2 > Threshold  OutDataTypeStr=fixdt_type_vsd
  VSD_6ph_30deg : MATLAB Function  TreatAsAtomicUnit=on
  alpha : Outport  OutDataTypeStr=fixdt(1,18,11)  VectorParamsAs1DForOutWhenUnconnected=off
  beta : Outport  Port=2  OutDataTypeStr=fixdt(1,18,11)  VectorParamsAs1DForOutWhenUnconnected=off
  x1 : Outport  Port=3  OutDataTypeStr=fixdt(1,18,11)  VectorParamsAs1DForOutWhenUnconnected=off
  y1 : Outport  Port=4  OutDataTypeStr=fixdt(1,18,11)  VectorParamsAs1DForOutWhenUnconnected=off
  z1 : Outport  Port=5  OutDataTypeStr=fixdt(1,18,11)  VectorParamsAs1DForOutWhenUnconnected=off
  z2 : Outport  Port=6  OutDataTypeStr=fixdt(1,18,11)  VectorParamsAs1DForOutWhenUnconnected=off
  vsd_done : Outport  Port=7  VectorParamsAs1DForOutWhenUnconnected=off
  alpha_AXI : Outport  Port=8  OutDataTypeStr=fixdt(1,18,11)  VectorParamsAs1DForOutWhenUnconnected=off
  beta_AXI : Outport  Port=9  OutDataTypeStr=fixdt(1,18,11)  VectorParamsAs1DForOutWhenUnconnected=off
  x_AXI : Outport  Port=10  OutDataTypeStr=fixdt(1,18,11)  VectorParamsAs1DForOutWhenUnconnected=off
  y_AXI : Outport  Port=11  OutDataTypeStr=fixdt(1,18,11)  VectorParamsAs1DForOutWhenUnconnected=off
  z1_AXI : Outport  Port=12  OutDataTypeStr=fixdt(1,18,11)  VectorParamsAs1DForOutWhenUnconnected=off
  z2_AXI : Outport  Port=13  OutDataTypeStr=fixdt(1,18,11)  VectorParamsAs1DForOutWhenUnconnected=off
  wires:
  VSD_6ph_30deg/1(alpha) -> Delay20/1, Delay14/1
  VSD_6ph_30deg/2(beta) -> Delay21/1, Delay15/1
  VSD_6ph_30deg/3(x1) -> Delay22/1, Delay16/1
  VSD_6ph_30deg/4(y1) -> Delay23/1, Delay17/1
  VSD_6ph_30deg/5(z1) -> Delay24/1, Delay18/1
  VSD_6ph_30deg/6(z2) -> Delay25/1, Delay19/1
  pu_conv_valid/1 -> Delay6/1
  Detect Rise Positive/1 -> Switch5/2, Switch4/2, Switch3/2, Switch2/2, Switch1/2, Switch/2, Delay13/1
  Delay/1 -> Switch/3
  Switch/1 -> VSD_6ph_30deg/1(a1), Delay/1
  Delay1/1 -> Switch1/3
  Switch1/1 -> VSD_6ph_30deg/2(b1), Delay1/1
  Delay2/1 -> Switch2/3
  Switch2/1 -> VSD_6ph_30deg/3(c1), Delay2/1
  Delay3/1 -> Switch3/3
  Switch3/1 -> VSD_6ph_30deg/4(a2), Delay3/1
  Delay4/1 -> Switch4/3
  Switch4/1 -> VSD_6ph_30deg/5(b2), Delay4/1
  Delay5/1 -> Switch5/3
  Switch5/1 -> VSD_6ph_30deg/6(c2), Delay5/1
  a1/1 -> Delay7/1
  b1/1 -> Delay8/1
  c1/1 -> Delay9/1
  a2/1 -> Delay10/1
  b2/1 -> Delay11/1
  c2/1 -> Delay12/1
  Delay6/1 -> Detect Rise Positive/1
  Delay7/1 -> Switch/1
  Delay8/1 -> Switch1/1
  Delay9/1 -> Switch2/1
  Delay10/1 -> Switch3/1
  Delay11/1 -> Switch4/1
  Delay12/1 -> Switch5/1
  Delay13/1 -> vsd_done/1
  Delay14/1 -> alpha/1
  Delay15/1 -> beta/1
  Delay16/1 -> x1/1
  Delay17/1 -> y1/1
  Delay18/1 -> z1/1
  Delay19/1 -> z2/1
  Delay20/1 -> alpha_AXI/1
  Delay21/1 -> beta_AXI/1
  Delay22/1 -> x_AXI/1
  Delay23/1 -> y_AXI/1
  Delay24/1 -> z1_AXI/1
  Delay25/1 -> z2_AXI/1

== matlab function uz_mpc_6ph/uz_vsd_6ph_30deg/VSD_6ph_30deg ==
  settings: fimath=fimath('RoundingMethod', 'Floor','OverflowAction', 'Wrap','ProductMode', 'FullPrecision', 'SumMode', 'FullPrecision')
  data: a1 input; alpha output; b1 input; c1 input; a2 input; b2 input; c2 input; beta output; x1 output; y1 output; z1 output; z2 output
function [alpha,beta,x1,y1,z1,z2] = fcn(a1,b1,c1,a2,b2,c2)


A = [fi(0,1,18,11) fi(0,1,18,11) fi(0,1,18,11) fi(0,1,18,11) fi(0,1,18,11) fi(0,1,18,11)]';

A =    2/6*[1    -0.5        -0.5        sqrt(3)/2   -sqrt(3)/2  0 ;
           0    sqrt(3)/2   -sqrt(3)/2  0.5         0.5         -1;
           1    -0.5        -0.5        -sqrt(3)/2  sqrt(3)/2   0 ;
           0    -sqrt(3)/2  sqrt(3)/2   0.5         0.5         -1;
           0.5   0.5          0.5          0           0           0 ;
           0    0           0           0.5          0.5          0.5] * [a1 b1 c1 a2 b2 c2]';

alpha = fi(A(1),1,18,11);
beta = fi(A(2),1,18,11);
x1 = fi(A(3),1,18,11);
y1 = fi(A(4),1,18,11);
z1 = fi(A(5),1,18,11);
z2 = fi(A(6),1,18,11);

== matlab function uz_mpc_6ph/prediciton ==
  settings: fimath=fimath('RoundingMethod', 'Floor','OverflowAction', 'Wrap','ProductMode', 'FullPrecision', 'SumMode', 'FullPrecision')
  data: vd_pu input; id_pred_pu output; vq_pu input; vx_pu input; vy_pu input; id_k_pu input; iq_k_pu input; ix_k_pu input; iy_k_pu input; omega_m_pu input; Ts_times_ZB_over_Ld input; Ts_times_ZB_over_Lq input; Ts_times_ZB_over_Lx input; Ts_times_ZB_over_Ly input; Rs_over_ZB input; Ld_over_LB input; Lq_over_LB input; psi_pm_over_psiB input; polepairs input; iq_pred_pu output; ix_pred_pu output; iy_pred_pu output
function [id_pred_pu,iq_pred_pu,ix_pred_pu,iy_pred_pu] = predict_currents(vd_pu,vq_pu,vx_pu,vy_pu,id_k_pu,iq_k_pu,ix_k_pu,iy_k_pu,...
                                                                                        omega_m_pu,Ts_times_ZB_over_Ld,Ts_times_ZB_over_Lq,...
                                                                                        Ts_times_ZB_over_Lx,Ts_times_ZB_over_Ly,Rs_over_ZB,Ld_over_LB,...
                                                                                        Lq_over_LB,psi_pm_over_psiB,polepairs)
    
                                                                                    
    fm = fimath();
    vd_pu = fi(vd_pu,1,27,24,fm);
    vq_pu = fi(vq_pu,1,27,24,fm);
    vx_pu = fi(vx_pu,1,27,24,fm);
    vy_pu = fi(vy_pu,1,27,24,fm);
    
    id_k_pu = fi(id_k_pu,1,27,16,fm);
    iq_k_pu = fi(iq_k_pu,1,27,16,fm);
    ix_k_pu = fi(ix_k_pu,1,27,16,fm);
    iy_k_pu = fi(iy_k_pu,1,27,16,fm);
    
    omega_m_pu = fi(omega_m_pu,1,18,15,fm);
    
    Ts_times_ZB_over_Ld = fi(Ts_times_ZB_over_Ld,1,18,15,fm);
    Ts_times_ZB_over_Lq = fi(Ts_times_ZB_over_Lq,1,18,15,fm);
    Ts_times_ZB_over_Lx = fi(Ts_times_ZB_over_Lx,1,18,15,fm);
    Ts_times_ZB_over_Ly = fi(Ts_times_ZB_over_Ly,1,18,15,fm);
    Rs_over_ZB = fi(Rs_over_ZB,1,18,15,fm);
    Ld_over_LB = fi(Ld_over_LB,1,18,15,fm);
    Lq_over_LB = fi(Lq_over_LB,1,18,15,fm);
    psi_pm_over_psiB = fi(psi_pm_over_psiB,1,18,15,fm);
    polepairs = fi(polepairs,0,18,0,fm);
                                                                                    
    num_switching_states = 64;
                                                                                    
    id_pred_pu = fi(zeros(num_switching_states,1),1,27,24,fm);
    iq_pred_pu = fi(zeros(num_switching_states,1),1,27,24,fm);
    ix_pred_pu = fi(zeros(num_switching_states,1),1,27,24,fm);
    iy_pred_pu = fi(zeros(num_switching_states,1),1,27,24,fm);
                                                                                        
    for i=1:num_switching_states                                                                            
                                                                                  
    %Prediction d-current
    id_pred_pu(i) = fi(Ts_times_ZB_over_Ld *(vd_pu(i) - Rs_over_ZB * id_k_pu + iq_k_pu * Lq_over_LB * omega_m_pu * polepairs) + id_k_pu,1,27,24);
    
    %Prediction q-current
    iq_pred_pu(i) = fi(Ts_times_ZB_over_Lq *(vq_pu(i) - Rs_over_ZB * iq_k_pu - omega_m_pu * polepairs * Ld_over_LB * id_k_pu - omega_m_pu * polepairs * psi_pm_over_psiB) + iq_k_pu,1,27,24);
       
    %Prediction x-current
    ix_pred_pu(i) = fi(Ts_times_ZB_over_Lx *(vx_pu(i) - Rs_over_ZB* ix_k_pu) + ix_k_pu,1,27,24);
   
    %Prediction y-current
    iy_pred_pu(i) = fi(Ts_times_ZB_over_Ly *(vy_pu(i) - Rs_over_ZB * iy_k_pu) + iy_k_pu,1,27,24);    
    
    end


end
